simulink model "Linear_n9960210"  (R2021a)
settings: Solver=VariableStepAuto  StartTime=0.0  StopTime=300  RelTol=1e-3
values from neighbouring files (symbols this model uses):
  A = [0 1 0 ... (first row only)    [main_n9960210_plotall.m]
  B = [0 ... (first row only)    [main_n9960210_plotall.m]
  C = [1 0 0]    [main_n9960210_plotall.m]
  L = place(A', C', p)'    [main_n9960210_plotall.m]
  u_bar = 1    [main_n9960210_plotall.m]
  use_state_variables = 1    [main_n9960210_plotall.m]
  x0 = [1.5 0 0]    [main_n9960210_plotall.m]
  x_bar = [2*u_bar-1 ... (first row only)    [main_n9960210_plotall.m]
undefined symbols (not defined in the file or in its folder): K
settings Model: Creator=isaac  LastModifiedBy=isaac

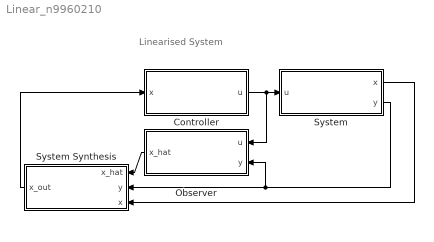
== system Linear_n9960210 ==
  note: Linearised System
  Controller : Subsystem
  Observer : Subsystem
  System : Subsystem
  System Synthesis : Subsystem
  wires:
  Controller/1(u) -> System/1(u), Observer/1(u)
  System/1(x) -> System Synthesis/3(x)
  System/2(y) -> System Synthesis/2(y), Observer/2(y)
  Observer/1(x_hat) -> System Synthesis/1(x_hat)
  System Synthesis/1(x_out) -> Controller/1(x)

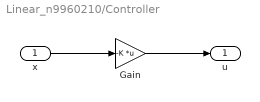
== system Linear_n9960210/Controller ==
  x : Inport
  Gain : Gain  Gain=-K  Multiplication=Matrix(K*u)
  u : Outport
  wires:
  Gain/1 -> u/1
  x/1 -> Gain/1

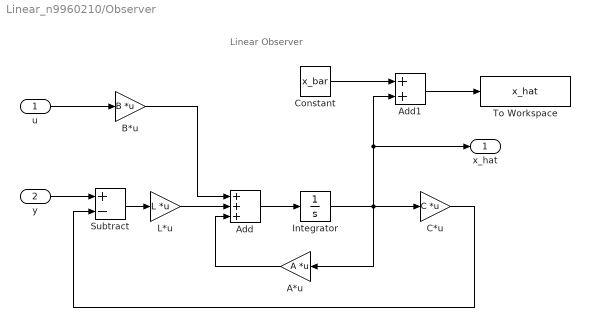
== system Linear_n9960210/Observer ==
  note: Linear Observer
  u : Inport
  y : Inport  Port=2
  A*u : Gain  Gain=A  Multiplication=Matrix(K*u)
  Add : Sum  Inputs=+++
  Add1 : Sum
  B*u : Gain  Gain=B  Multiplication=Matrix(K*u)
  C*u : Gain  Gain=C  Multiplication=Matrix(K*u)
  Constant : Constant  Value=x_bar
  Integrator : Integrator  InitialCondition=x0-x_bar'
  L*u : Gain  Gain=L  Multiplication=Matrix(K*u)
  Subtract : Sum  Inputs=+-
  To Workspace : ToWorkspace  VariableName=x_hat  SampleTime=-1
  x_hat : Outport
  wires:
  L*u/1 -> Add/2
  Add/1 -> Integrator/1
  A*u/1 -> Add/3
  Constant/1 -> Add1/1
  y/1 -> Subtract/1
  Subtract/1 -> L*u/1
  Add1/1 -> To Workspace/1
  Integrator/1 -> x_hat/1, Add1/2, C*u/1, A*u/1
  C*u/1 -> Subtract/2
  B*u/1 -> Add/1
  u/1 -> B*u/1

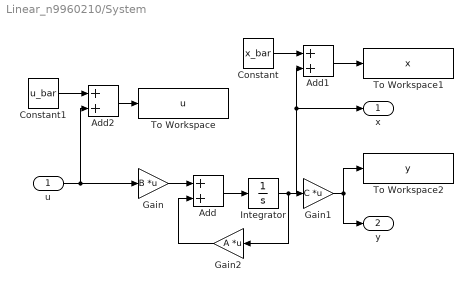
== system Linear_n9960210/System ==
  u : Inport
  Add : Sum
  Add1 : Sum
  Add2 : Sum
  Constant : Constant  Value=x_bar
  Constant1 : Constant  Value=u_bar
  Gain : Gain  Gain=B  Multiplication=Matrix(K*u)
  Gain1 : Gain  Gain=C  Multiplication=Matrix(K*u)
  Gain2 : Gain  Gain=A  Multiplication=Matrix(K*u)
  Integrator : Integrator  InitialCondition=x0-x_bar'
  To Workspace : ToWorkspace  VariableName=u  SampleTime=-1
  To Workspace1 : ToWorkspace  VariableName=x  SampleTime=-1
  To Workspace2 : ToWorkspace  VariableName=y  SampleTime=-1
  x : Outport
  y : Outport  Port=2
  wires:
  u/1 -> Add2/2, Gain/1
  Gain/1 -> Add/1
  Add/1 -> Integrator/1
  Gain2/1 -> Add/2
  Gain1/1 -> y/1, To Workspace2/1
  Constant/1 -> Add1/1
  Integrator/1 -> Add1/2, x/1, Gain2/1, Gain1/1
  Add1/1 -> To Workspace1/1
  Add2/1 -> To Workspace/1
  Constant1/1 -> Add2/1

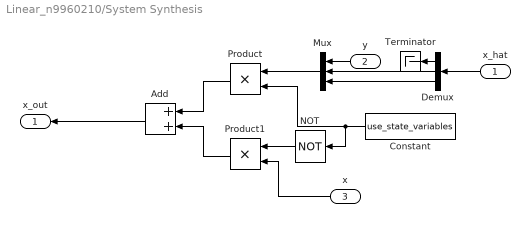
== system Linear_n9960210/System Synthesis ==
  x_hat : Inport
  y : Inport  Port=2
  x : Inport  Port=3
  Add : Sum
  Constant : Constant  Value=use_state_variables
  Demux : Demux  Outputs=3
  Mux : Mux  Inputs=3
  NOT : Logic  Operator=NOT  IconShape=distinctive  AllPortsSameDT=off  OutDataTypeStr=boolean
  Product : Product
  Product1 : Product
  Terminator : Terminator
  x_out : Outport
  wires:
  Product/1 -> Add/1
  Product1/1 -> Add/2
  NOT/1 -> Product1/1
  Constant/1 -> Product/2, NOT/1
  x/1 -> Product1/2
  x_hat/1 -> Demux/1
  Demux/3 -> Mux/3
  Add/1 -> x_out/1
  Mux/1 -> Product/1
  Demux/2 -> Mux/2
  Demux/1 -> Terminator/1
  y/1 -> Mux/1
